simulink model "AXI_QPSK_Rx"  (R2017b)
settings: Solver=VariableStepAuto  StartTime=0.0  StopTime=2500/Rb  RelTol=1e-3
PreLoadFcn:
  | design_filters_rx;      % run script to generate filter designs.
  | 
  | Rb = 1000;   % 1kbit / s
  | 
  | Rsym = Rb/2;   % 2 bits per symbol
  | 
  | Rsymbol = Rb/2;
  | 
  | OSR = 32;
  | 
  | f_error = 120;
  | 
  | fc = 100e3;
values from neighbouring files (symbols this model uses):
  CIC_fine_Rx = 2^(-(CIC_right_shift_i-CIC_shift_Rx))    [design_filters_rx.m]
  fCIC = fCICcomp * R_CIC    (= 25600000)    [design_filters_rx.m]
  R_CIC = 3200    [design_filters_rx.m]
  R_CICcomp = 2    [design_filters_rx.m]
  R_HB = 2    [design_filters_rx.m]
  R_RRC = 4    [design_filters_rx.m]
undefined symbols (not defined in the file or in its folder): AXI4, designMultirateFIR, Lite
libraries: xbsIndex_r4 x539, dspmlti4 x12, dsparch4 x2, dspsrcs4 x2, commrandsrc2 x1, commdigbbndpm3 x1
(part 2 of 5)

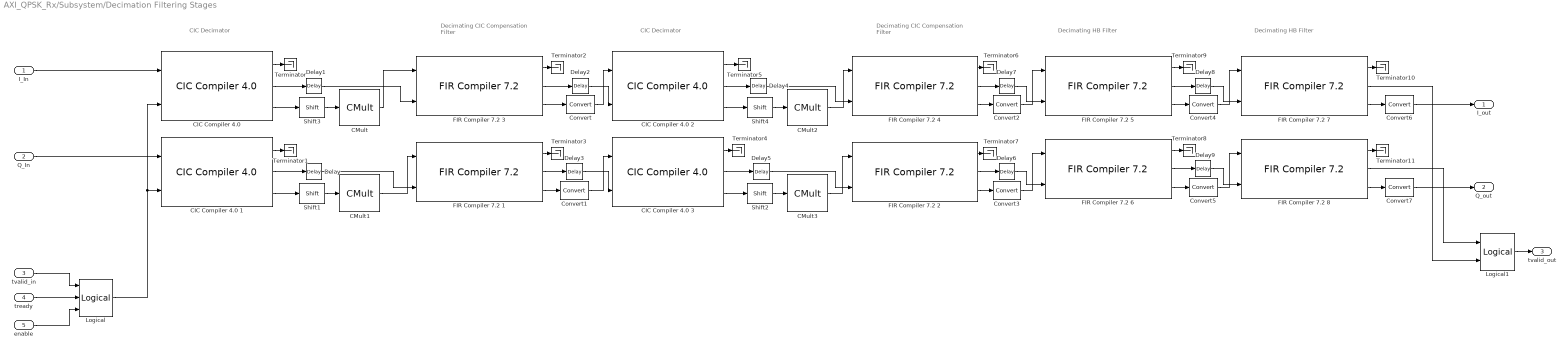
== system AXI_QPSK_Rx/Subsystem/Decimation Filtering Stages ==
  note: CIC Decimator
  note: Decimating CIC
      | Compensation Filter
  note: CIC Decimator
  note: Decimating CIC
      | Compensation Filter
  note: Decimating HB Filter
  note: Decimating HB Filter
  I_In : Inport
  Q_In : Inport  Port=2
  tvalid_in : Inport  Port=3
  tready : Inport  Port=4
  enable : Inport  Port=5
  CIC Compiler 4.0 {,1..3} (4 alike) : xbsIndex_r4/CIC Compiler 4.0   filter_type=Decimation  number_of_stages=3  differential_delay=1  number_of_channels=1  sample_rate_changes=Fixed  fixed_or_initial_rate=R_CIC_i  minimum_rate=20  maximum_rate=20  ratespecification=Maximum_Possible  sampleperiod=1  hardwareoversamplingrate=1  quantization=Full_Precision  output_data_width=31  use_xtreme_dsp_slice=on  use_streaming_interface=on  has_aclken=on  has_aresetn=off  has_dout_tready=off  trim_axipin_name=on  gui_behaviour=Sysgen_GUI  input_data_width=18  ip_name=CIC Compiler  ip_version=4.0  dsptool_ready=true  wrapper_available=true  port_translation_map={ 'aclken' => 'en', 'aresetn' => 'rst' }  ipcore_xco_need_fpga_part=true  ipcore_verbose=false  block_type=cic_compiler_v4_0
  CMult{,1..3} (4 alike) : xbsIndex_r4/CMult  const=CIC_fine_Rx  gui_display_data_type=Fixed-point  const_n_bits=16  const_bin_pt=14  float_type=Single  exp_bits=8  fraction_bits=24  en=off  latency=1  precision=User Defined  arith_type="Signed  (2's comp)"  n_bits=16  bin_pt=14  quantization=Truncate  overflow=Wrap  use_behavioral_HDL=off  mem_type=Distributed RAM  pipeline=off  dbl_ovrd=off  block_type=cmult
  Convert{,1..7} (8 alike) : xbsIndex_r4/Convert  gui_display_data_type=Fixed-point  arith_type="Signed  (2's comp)"  n_bits=16  bin_pt=14  float_type=Single  exp_bits=8  fraction_bits=24  quantization=Truncate  overflow=Wrap  en=off  latency=1  pipeline=off  dbl_ovrd=off  block_type=convert
  Delay{,1..9} (10 alike) : xbsIndex_r4/Delay  rst=off  infoeditControl=Selection of Reset will increase slice count due to use of real FFs and instead of SRLs  en=off  latency=1  reg_retiming=off  dbl_ovrd=off  block_type=delay
  FIR Compiler 7.2 {1..4} (4 alike) : xbsIndex_r4/FIR Compiler 7.2   coefficientvector=WComp_i.Numerator  coefficient_sets=1  coefficient_reload=off  filter_type=Decimation  rate_change_type=Integer  interpolation_rate=1  decimation_rate=2  zero_pack_factor=1  channel_sequence=Basic  number_channels=1  pattern_list='P4-0,P4-1,P4-2,P4-3,P4-4'  number_paths=1  ratespecification=Maximum_Possible  sampleperiod=3200  hardwareoversamplingrate=1  coefficient_sign=Signed  quantization=Quantize_Only  coefficient_width=16  bestprecision=on  coefficient_fractional_bits=15  coefficient_structure=Inferred  output_rounding_mode=Full_Precision  output_width=33  filter_architecture=Systolic_Multiply_Accumulate  optimization_goal=Area  optimization_list='None'  data_buffer_type=Automatic  coefficient_buffer_type=Automatic  input_buffer_type=Automatic  output_buffer_type=Automatic  preference_for_other_storage=Automatic  multi_column_support=Automatic  columnconfig='10'  inter_column_pipe_length=4  data_has_tlast=Not_Required  m_data_has_tready=off  s_data_has_fifo=off  s_data_has_tuser=Not_Required  m_data_has_tuser=Not_Required  s_config_sync_mode=On_Vector  s_config_method=Single  num_reload_slots=1  has_aclken=on  has_aresetn=off  infoeditControl=ARESETn must be asserted for a minimum of 2 cycles  reset_data_vector=on  trim_axipin_name=on  simulation_type=hybrid_sim  simulation_model=sysgen:xfirv7_2_cmodel  data_path_portlist={ 's_axis_data_tdata', 'm_axis_data_tdata' }  passband_min=0.0  passband_max=0.5  stopband_min=0.5  stopband_max=1.0  filter_selection=1  gui_behaviour='Sysgen_GUI'  data_sign=Signed  data_width=16  data_fractional_bits=0  data_tuser_width=1  wrapper_available=true  ip_wrap_arbitrary_binary_point=true  ip_name=FIR Compiler  ip_version=7.2  dsptool_ready=true  ipcore_usecache=true  ipcore_useipmodelcache=true  port_translation_map={ 'aclken' => 'en', 'aresetn' => 'rst' }  run_core_at_system_period=true  ipcore_xco_need_fpga_part=true  block_type=fir_compiler_v7_2
      settings: infoedit=Maximum Possible : Maximizes oversampling rate. Abstracted input handshake (no s_data_tvalid) and automatic rate propagation.<br>Hardware Oversampling Rate : Specifies oversampling rate relative to the input sample period. Abstracted input handshake (no s_data_tvalid) and automatic rate propagation.<br>Input/Output Sample Period : Specifies absolute oversampling rate. No input handshake abstraction (exposes s_data_tvalid) and no rate propagation.
  FIR Compiler 7.2 {5..8} (4 alike) : xbsIndex_r4/FIR Compiler 7.2   coefficientvector=HB.Numerator  coefficient_sets=1  coefficient_reload=off  filter_type=Decimation  rate_change_type=Integer  interpolation_rate=1  decimation_rate=2  zero_pack_factor=1  channel_sequence=Basic  number_channels=1  pattern_list='P4-0,P4-1,P4-2,P4-3,P4-4'  number_paths=1  ratespecification=Maximum_Possible  sampleperiod=3200  hardwareoversamplingrate=1  coefficient_sign=Signed  quantization=Quantize_Only  coefficient_width=16  bestprecision=on  coefficient_fractional_bits=15  coefficient_structure=Inferred  output_rounding_mode=Full_Precision  output_width=32  filter_architecture=Systolic_Multiply_Accumulate  optimization_goal=Area  optimization_list='None'  data_buffer_type=Automatic  coefficient_buffer_type=Automatic  input_buffer_type=Automatic  output_buffer_type=Automatic  preference_for_other_storage=Automatic  multi_column_support=Automatic  columnconfig='6'  inter_column_pipe_length=4  data_has_tlast=Not_Required  m_data_has_tready=off  s_data_has_fifo=off  s_data_has_tuser=Not_Required  m_data_has_tuser=Not_Required  s_config_sync_mode=On_Vector  s_config_method=Single  num_reload_slots=1  has_aclken=on  has_aresetn=off  infoeditControl=ARESETn must be asserted for a minimum of 2 cycles  reset_data_vector=on  trim_axipin_name=on  simulation_type=hybrid_sim  simulation_model=sysgen:xfirv7_2_cmodel  data_path_portlist={ 's_axis_data_tdata', 'm_axis_data_tdata' }  passband_min=0.0  passband_max=0.5  stopband_min=0.5  stopband_max=1.0  filter_selection=1  gui_behaviour='Sysgen_GUI'  data_sign=Signed  data_width=16  data_fractional_bits=0  data_tuser_width=1  wrapper_available=true  ip_wrap_arbitrary_binary_point=true  ip_name=FIR Compiler  ip_version=7.2  dsptool_ready=true  ipcore_usecache=true  ipcore_useipmodelcache=true  port_translation_map={ 'aclken' => 'en', 'aresetn' => 'rst' }  run_core_at_system_period=true  ipcore_xco_need_fpga_part=true  block_type=fir_compiler_v7_2
      settings: infoedit=Maximum Possible : Maximizes oversampling rate. Abstracted input handshake (no s_data_tvalid) and automatic rate propagation.<br>Hardware Oversampling Rate : Specifies oversampling rate relative to the input sample period. Abstracted input handshake (no s_data_tvalid) and automatic rate propagation.<br>Input/Output Sample Period : Specifies absolute oversampling rate. No input handshake abstraction (exposes s_data_tvalid) and no rate propagation.
  Logical : xbsIndex_r4/Logical  logical_function=AND  inputs=3  en=off  latency=0  precision=Full  arith_type=Unsigned  n_bits=16  bin_pt=0  align_bp=on  dbl_ovrd=off  block_type=logical
  Logical1 : xbsIndex_r4/Logical  logical_function=AND  inputs=2  en=off  latency=1  precision=Full  arith_type=Unsigned  n_bits=16  bin_pt=0  align_bp=on  dbl_ovrd=off  block_type=logical
  Shift{1..4} (4 alike) : xbsIndex_r4/Shift  shift_dir=Right  shift_bits=CIC_shift_Rx  en=off  latency=0  precision=User Defined  arith_type="Signed  (2's comp)"  n_bits=17  bin_pt=14  quantization=Truncate  overflow=Wrap  dbl_ovrd=off  block_type=shift
  Terminator{,1..11} (12 alike) : Terminator
  I_out : Outport
  Q_out : Outport  Port=2
  tvalid_out : Outport  Port=3
  wires:
  FIR Compiler 7.2 1/3 -> Convert1/1
  Shift1/1 -> CMult1/1
  CIC Compiler 4.0 1/3 -> Shift1/1
  "CIC Compiler 4.0 "/3 -> Shift3/1
  Shift3/1 -> CMult/1
  FIR Compiler 7.2 3/3 -> Convert/1
  CMult/1 -> FIR Compiler 7.2 3/1
  CMult1/1 -> FIR Compiler 7.2 1/1
  CMult3/1 -> FIR Compiler 7.2 2/1
  CMult2/1 -> FIR Compiler 7.2 4/1
  FIR Compiler 7.2 4/3 -> Convert2/1
  Shift4/1 -> CMult2/1
  CIC Compiler 4.0 2/3 -> Shift4/1
  CIC Compiler 4.0 3/3 -> Shift2/1
  Shift2/1 -> CMult3/1
  FIR Compiler 7.2 2/3 -> Convert3/1
  Convert/1 -> CIC Compiler 4.0 2/1
  Convert1/1 -> CIC Compiler 4.0 3/1
  Convert2/1 -> FIR Compiler 7.2 5/1
  Convert3/1 -> FIR Compiler 7.2 6/1
  FIR Compiler 7.2 6/3 -> Convert5/1
  FIR Compiler 7.2 5/3 -> Convert4/1
  Convert4/1 -> FIR Compiler 7.2 7/1
  Convert5/1 -> FIR Compiler 7.2 8/1
  FIR Compiler 7.2 7/3 -> Convert6/1
  FIR Compiler 7.2 8/3 -> Convert7/1
  Convert6/1 -> I_out/1
  Convert7/1 -> Q_out/1
  tready/1 -> Logical/2
  tvalid_in/1 -> Logical/1
  enable/1 -> Logical/3
  Logical/1 -> CIC Compiler 4.0 1/2, "CIC Compiler 4.0 "/2
  CIC Compiler 4.0 1/2 -> Delay/1
  Delay/1 -> FIR Compiler 7.2 1/2
  "CIC Compiler 4.0 "/2 -> Delay1/1
  Delay1/1 -> FIR Compiler 7.2 3/2
  FIR Compiler 7.2 3/2 -> Delay2/1
  Delay2/1 -> CIC Compiler 4.0 2/2
  FIR Compiler 7.2 1/2 -> Delay3/1
  Delay3/1 -> CIC Compiler 4.0 3/2
  CIC Compiler 4.0 2/2 -> Delay4/1
  Delay4/1 -> FIR Compiler 7.2 4/2
  CIC Compiler 4.0 3/2 -> Delay5/1
  Delay5/1 -> FIR Compiler 7.2 2/2
  FIR Compiler 7.2 2/2 -> Delay6/1
  Delay6/1 -> FIR Compiler 7.2 6/2
  FIR Compiler 7.2 4/2 -> Delay7/1
  Delay7/1 -> FIR Compiler 7.2 5/2
  FIR Compiler 7.2 5/2 -> Delay8/1
  Delay8/1 -> FIR Compiler 7.2 7/2
  FIR Compiler 7.2 6/2 -> Delay9/1
  Delay9/1 -> FIR Compiler 7.2 8/2
  Logical1/1 -> tvalid_out/1
  "CIC Compiler 4.0 "/1 -> Terminator/1
  CIC Compiler 4.0 1/1 -> Terminator1/1
  FIR Compiler 7.2 3/1 -> Terminator2/1
  FIR Compiler 7.2 1/1 -> Terminator3/1
  CIC Compiler 4.0 3/1 -> Terminator4/1
  CIC Compiler 4.0 2/1 -> Terminator5/1
  FIR Compiler 7.2 4/1 -> Terminator6/1
  FIR Compiler 7.2 2/1 -> Terminator7/1
  FIR Compiler 7.2 6/1 -> Terminator8/1
  FIR Compiler 7.2 5/1 -> Terminator9/1
  FIR Compiler 7.2 7/1 -> Terminator10/1
  FIR Compiler 7.2 8/2 -> Logical1/1
  FIR Compiler 7.2 7/2 -> Logical1/2
  FIR Compiler 7.2 8/1 -> Terminator11/1
  I_In/1 -> "CIC Compiler 4.0 "/1
  Q_In/1 -> CIC Compiler 4.0 1/1

== system AXI_QPSK_Rx/Subsystem/M_AXIS ==
  tData_in : Inport
  tValid_in : Inport  Port=2
  tLast_in : Inport  Port=3
  tReady_in : Inport  Port=4
  m_rf_axis_tdata : xbsIndex_r4/Gateway Out  inherit_from_input=off  hdl_port=on  rows=1  columns=1  UseAsDAC=off  DACChannel='1'  interface=None  automatic_assignment=on  address_offset=hex2dec('00')  intf_name=''  intf_description=''  timing_constraint=None  locs_specified=off  LOCs={}  io_standard={}  block_type=gatewayout
  m_rf_axis_tlast : xbsIndex_r4/Gateway Out  inherit_from_input=off  hdl_port=on  rows=1  columns=1  UseAsDAC=off  DACChannel='1'  interface=None  automatic_assignment=on  address_offset=hex2dec('00')  intf_name=''  intf_description=''  timing_constraint=None  locs_specified=off  LOCs={}  io_standard={}  block_type=gatewayout
  m_rf_axis_tready : xbsIndex_r4/Gateway In  gui_display_data_type=Boolean  arith_type=Boolean  n_bits=16  bin_pt=14  preci_type=Single  exp_width=8  frac_width=24  rows=1  columns=1  quantization="Round  (unbiased: +/- Inf)"  overflow=Saturate  period=1/(0.5*R_RRC*R_HB*R_CICcomp*R_CIC*Rb)  UseAsADC=off  ADCChannel='1'  interface=None  automatic_assignment=on  address_offset=hex2dec('00')  intf_name=''  intf_description=''  default_value=0  timing_constraint=None  locs_specified=off  LOCs={}  io_standard={}  inherit_from_input=off  hdl_port=on  dbl_ovrd=off  block_type=gatewayin
  m_rf_axis_tvalid : xbsIndex_r4/Gateway Out  inherit_from_input=off  hdl_port=on  rows=1  columns=1  UseAsDAC=off  DACChannel='1'  interface=None  automatic_assignment=on  address_offset=hex2dec('00')  intf_name=''  intf_description=''  timing_constraint=None  locs_specified=off  LOCs={}  io_standard={}  block_type=gatewayout
  tData_out : Outport
  tLast_out : Outport  Port=2
  tValid_out : Outport  Port=3
  tReady_out : Outport  Port=4
  wires:
  tReady_in/1 -> m_rf_axis_tready/1
  m_rf_axis_tlast/1 -> tLast_out/1
  m_rf_axis_tvalid/1 -> tValid_out/1
  m_rf_axis_tdata/1 -> tData_out/1
  tData_in/1 -> m_rf_axis_tdata/1
  tLast_in/1 -> m_rf_axis_tlast/1
  tValid_in/1 -> m_rf_axis_tvalid/1
  m_rf_axis_tready/1 -> tReady_out/1

== system AXI_QPSK_Rx/Subsystem/M_AXIS_DECIMATION ==
  tData_in : Inport
  tValid_in : Inport  Port=2
  tLast_in : Inport  Port=3
  tReady_in : Inport  Port=4
  m_dec_axis_tdata : xbsIndex_r4/Gateway Out  inherit_from_input=off  hdl_port=on  rows=1  columns=1  UseAsDAC=off  DACChannel='1'  interface=None  automatic_assignment=on  address_offset=hex2dec('00')  intf_name=''  intf_description=''  timing_constraint=None  locs_specified=off  LOCs={}  io_standard={}  block_type=gatewayout
  m_dec_axis_tlast : xbsIndex_r4/Gateway Out  inherit_from_input=off  hdl_port=on  rows=1  columns=1  UseAsDAC=off  DACChannel='1'  interface=None  automatic_assignment=on  address_offset=hex2dec('00')  intf_name=''  intf_description=''  timing_constraint=None  locs_specified=off  LOCs={}  io_standard={}  block_type=gatewayout
  m_dec_axis_tready : xbsIndex_r4/Gateway In  gui_display_data_type=Boolean  arith_type=Boolean  n_bits=16  bin_pt=14  preci_type=Single  exp_width=8  frac_width=24  rows=1  columns=1  quantization="Round  (unbiased: +/- Inf)"  overflow=Saturate  period=1/(0.5*R_RRC*R_HB*R_CICcomp*R_CIC*Rb)  UseAsADC=off  ADCChannel='1'  interface=None  automatic_assignment=on  address_offset=hex2dec('00')  intf_name=''  intf_description=''  default_value=0  timing_constraint=None  locs_specified=off  LOCs={}  io_standard={}  inherit_from_input=off  hdl_port=on  dbl_ovrd=off  block_type=gatewayin
  m_dec_axis_tvalid : xbsIndex_r4/Gateway Out  inherit_from_input=off  hdl_port=on  rows=1  columns=1  UseAsDAC=off  DACChannel='1'  interface=None  automatic_assignment=on  address_offset=hex2dec('00')  intf_name=''  intf_description=''  timing_constraint=None  locs_specified=off  LOCs={}  io_standard={}  block_type=gatewayout
  tData_out : Outport
  tLast_out : Outport  Port=2
  tValid_out : Outport  Port=3
  tReady_out : Outport  Port=4
  wires:
  m_dec_axis_tready/1 -> tReady_out/1
  tValid_in/1 -> m_dec_axis_tvalid/1
  tLast_in/1 -> m_dec_axis_tlast/1
  tData_in/1 -> m_dec_axis_tdata/1
  m_dec_axis_tdata/1 -> tData_out/1
  m_dec_axis_tvalid/1 -> tValid_out/1
  m_dec_axis_tlast/1 -> tLast_out/1
  tReady_in/1 -> m_dec_axis_tready/1

== system AXI_QPSK_Rx/Subsystem/M_AXIS_FREQ_SYNC ==
  tData_in : Inport
  tValid_in : Inport  Port=2
  tLast_in : Inport  Port=3
  tReady_in : Inport  Port=4
  m_sync_axis_tdata : xbsIndex_r4/Gateway Out  inherit_from_input=off  hdl_port=on  rows=1  columns=1  UseAsDAC=off  DACChannel='1'  interface=None  automatic_assignment=on  address_offset=hex2dec('00')  intf_name=''  intf_description=''  timing_constraint=None  locs_specified=off  LOCs={}  io_standard={}  block_type=gatewayout
  m_sync_axis_tlast : xbsIndex_r4/Gateway Out  inherit_from_input=off  hdl_port=on  rows=1  columns=1  UseAsDAC=off  DACChannel='1'  interface=None  automatic_assignment=on  address_offset=hex2dec('00')  intf_name=''  intf_description=''  timing_constraint=None  locs_specified=off  LOCs={}  io_standard={}  block_type=gatewayout
  m_sync_axis_tready : xbsIndex_r4/Gateway In  gui_display_data_type=Boolean  arith_type=Boolean  n_bits=16  bin_pt=14  preci_type=Single  exp_width=8  frac_width=24  rows=1  columns=1  quantization="Round  (unbiased: +/- Inf)"  overflow=Saturate  period=1/(0.5*R_RRC*R_HB*R_CICcomp*R_CIC*Rb)  UseAsADC=off  ADCChannel='1'  interface=None  automatic_assignment=on  address_offset=hex2dec('00')  intf_name=''  intf_description=''  default_value=0  timing_constraint=None  locs_specified=off  LOCs={}  io_standard={}  inherit_from_input=off  hdl_port=on  dbl_ovrd=off  block_type=gatewayin
  m_sync_axis_tvalid : xbsIndex_r4/Gateway Out  inherit_from_input=off  hdl_port=on  rows=1  columns=1  UseAsDAC=off  DACChannel='1'  interface=None  automatic_assignment=on  address_offset=hex2dec('00')  intf_name=''  intf_description=''  timing_constraint=None  locs_specified=off  LOCs={}  io_standard={}  block_type=gatewayout
  tData_out : Outport
  tLast_out : Outport  Port=2
  tValid_out : Outport  Port=3
  tReady_out : Outport  Port=4
  wires:
  tReady_in/1 -> m_sync_axis_tready/1
  m_sync_axis_tlast/1 -> tLast_out/1
  m_sync_axis_tvalid/1 -> tValid_out/1
  m_sync_axis_tdata/1 -> tData_out/1
  tData_in/1 -> m_sync_axis_tdata/1
  tLast_in/1 -> m_sync_axis_tlast/1
  tValid_in/1 -> m_sync_axis_tvalid/1
  m_sync_axis_tready/1 -> tReady_out/1

== system AXI_QPSK_Rx/Subsystem/M_AXIS_RRC ==
  tData_in : Inport
  tValid_in : Inport  Port=2
  tLast_in : Inport  Port=3
  tReady_in : Inport  Port=4
  m_rrc_axis_tdata : xbsIndex_r4/Gateway Out  inherit_from_input=off  hdl_port=on  rows=1  columns=1  UseAsDAC=off  DACChannel='1'  interface=None  automatic_assignment=on  address_offset=hex2dec('00')  intf_name=''  intf_description=''  timing_constraint=None  locs_specified=off  LOCs={}  io_standard={}  block_type=gatewayout
  m_rrc_axis_tlast : xbsIndex_r4/Gateway Out  inherit_from_input=off  hdl_port=on  rows=1  columns=1  UseAsDAC=off  DACChannel='1'  interface=None  automatic_assignment=on  address_offset=hex2dec('00')  intf_name=''  intf_description=''  timing_constraint=None  locs_specified=off  LOCs={}  io_standard={}  block_type=gatewayout
  m_rrc_axis_tready : xbsIndex_r4/Gateway In  gui_display_data_type=Boolean  arith_type=Boolean  n_bits=16  bin_pt=14  preci_type=Single  exp_width=8  frac_width=24  rows=1  columns=1  quantization="Round  (unbiased: +/- Inf)"  overflow=Saturate  period=1/(0.5*R_RRC*R_HB*R_CICcomp*R_CIC*Rb)  UseAsADC=off  ADCChannel='1'  interface=None  automatic_assignment=on  address_offset=hex2dec('00')  intf_name=''  intf_description=''  default_value=0  timing_constraint=None  locs_specified=off  LOCs={}  io_standard={}  inherit_from_input=off  hdl_port=on  dbl_ovrd=off  block_type=gatewayin
  m_rrc_axis_tvalid : xbsIndex_r4/Gateway Out  inherit_from_input=off  hdl_port=on  rows=1  columns=1  UseAsDAC=off  DACChannel='1'  interface=None  automatic_assignment=on  address_offset=hex2dec('00')  intf_name=''  intf_description=''  timing_constraint=None  locs_specified=off  LOCs={}  io_standard={}  block_type=gatewayout
  tData_out : Outport
  tLast_out : Outport  Port=2
  tValid_out : Outport  Port=3
  tReady_out : Outport  Port=4
  wires:
  tReady_in/1 -> m_rrc_axis_tready/1
  m_rrc_axis_tlast/1 -> tLast_out/1
  m_rrc_axis_tvalid/1 -> tValid_out/1
  m_rrc_axis_tdata/1 -> tData_out/1
  tData_in/1 -> m_rrc_axis_tdata/1
  tLast_in/1 -> m_rrc_axis_tlast/1
  tValid_in/1 -> m_rrc_axis_tvalid/1
  m_rrc_axis_tready/1 -> tReady_out/1

== system AXI_QPSK_Rx/Subsystem/RRC Filtering and Pre-Synch Interpolation  ==
  note: Root Raised Cosine Receive Filter
      | (single rate)
  note: Interpolating (x2) Halfband Filter
  note: Interpolating (x2) Halfband Filter
  I_in : Inport
  Q_in : Inport  Port=2
  tvalid_in : Inport  Port=3
  Delay{1..4} (4 alike) : xbsIndex_r4/Delay  rst=off  infoeditControl=Selection of Reset will increase slice count due to use of real FFs and instead of SRLs  en=off  latency=1  reg_retiming=off  dbl_ovrd=off  block_type=delay
  FIR Compiler 7.2 2 : xbsIndex_r4/FIR Compiler 7.2   coefficientvector=WRRC2.Numerator  coefficient_sets=1  coefficient_reload=off  filter_type=Single_Rate  rate_change_type=Integer  interpolation_rate=1  decimation_rate=1  zero_pack_factor=1  channel_sequence=Basic  number_channels=1  pattern_list='P4-0,P4-1,P4-2,P4-3,P4-4'  number_paths=1  ratespecification=Maximum_Possible  sampleperiod=1  hardwareoversamplingrate=1  coefficient_sign=Signed  quantization=Quantize_Only  coefficient_width=16  bestprecision=on  coefficient_fractional_bits=16  coefficient_structure=Inferred  output_rounding_mode=Full_Precision  output_width=35  filter_architecture=Systolic_Multiply_Accumulate  optimization_goal=Area  optimization_list='None'  data_buffer_type=Automatic  coefficient_buffer_type=Automatic  input_buffer_type=Automatic  output_buffer_type=Automatic  preference_for_other_storage=Automatic  multi_column_support=Automatic  columnconfig='49'  inter_column_pipe_length=4  data_has_tlast=Not_Required  m_data_has_tready=off  s_data_has_fifo=off  s_data_has_tuser=Not_Required  m_data_has_tuser=Not_Required  s_config_sync_mode=On_Vector  s_config_method=Single  num_reload_slots=1  has_aclken=on  has_aresetn=off  infoeditControl=ARESETn must be asserted for a minimum of 2 cycles  reset_data_vector=on  trim_axipin_name=on  simulation_type=hybrid_sim  simulation_model=sysgen:xfirv7_2_cmodel  data_path_portlist={ 's_axis_data_tdata', 'm_axis_data_tdata' }  passband_min=0.0  passband_max=0.5  stopband_min=0.5  stopband_max=1.0  filter_selection=1  gui_behaviour='Sysgen_GUI'  data_sign=Signed  data_width=16  data_fractional_bits=0  data_tuser_width=1  wrapper_available=true  ip_wrap_arbitrary_binary_point=true  ip_name=FIR Compiler  ip_version=7.2  dsptool_ready=true  ipcore_usecache=true  ipcore_useipmodelcache=true  port_translation_map={ 'aclken' => 'en', 'aresetn' => 'rst' }  run_core_at_system_period=true  ipcore_xco_need_fpga_part=true  block_type=fir_compiler_v7_2
      settings: infoedit=Maximum Possible : Maximizes oversampling rate. Abstracted input handshake (no s_data_tvalid) and automatic rate propagation.<br>Hardware Oversampling Rate : Specifies oversampling rate relative to the input sample period. Abstracted input handshake (no s_data_tvalid) and automatic rate propagation.<br>Input/Output Sample Period : Specifies absolute oversampling rate. No input handshake abstraction (exposes s_data_tvalid) and no rate propagation.
  FIR Compiler 7.2 4 : xbsIndex_r4/FIR Compiler 7.2   coefficientvector=WRRC2.Numerator  coefficient_sets=1  coefficient_reload=off  filter_type=Single_Rate  rate_change_type=Integer  interpolation_rate=1  decimation_rate=1  zero_pack_factor=1  channel_sequence=Basic  number_channels=1  pattern_list='P4-0,P4-1,P4-2,P4-3,P4-4'  number_paths=1  ratespecification=Maximum_Possible  sampleperiod=1  hardwareoversamplingrate=1  coefficient_sign=Signed  quantization=Quantize_Only  coefficient_width=16  bestprecision=on  coefficient_fractional_bits=16  coefficient_structure=Inferred  output_rounding_mode=Full_Precision  output_width=35  filter_architecture=Systolic_Multiply_Accumulate  optimization_goal=Area  optimization_list='None'  data_buffer_type=Automatic  coefficient_buffer_type=Automatic  input_buffer_type=Automatic  output_buffer_type=Automatic  preference_for_other_storage=Automatic  multi_column_support=Automatic  columnconfig='49'  inter_column_pipe_length=4  data_has_tlast=Not_Required  m_data_has_tready=off  s_data_has_fifo=off  s_data_has_tuser=Not_Required  m_data_has_tuser=Not_Required  s_config_sync_mode=On_Vector  s_config_method=Single  num_reload_slots=1  has_aclken=on  has_aresetn=off  infoeditControl=ARESETn must be asserted for a minimum of 2 cycles  reset_data_vector=on  trim_axipin_name=on  simulation_type=hybrid_sim  simulation_model=sysgen:xfirv7_2_cmodel  data_path_portlist={ 's_axis_data_tdata', 'm_axis_data_tdata' }  passband_min=0.0  passband_max=0.5  stopband_min=0.5  stopband_max=1.0  filter_selection=1  gui_behaviour='Sysgen_GUI'  data_sign=Signed  data_width=16  data_fractional_bits=0  data_tuser_width=1  wrapper_available=true  ip_wrap_arbitrary_binary_point=true  ip_name=FIR Compiler  ip_version=7.2  dsptool_ready=true  ipcore_usecache=true  ipcore_useipmodelcache=true  port_translation_map={ 'aclken' => 'en', 'aresetn' => 'rst' }  run_core_at_system_period=true  ipcore_xco_need_fpga_part=true  block_type=fir_compiler_v7_2
      settings: infoedit=Maximum Possible : Maximizes oversampling rate. Abstracted input handshake (no s_data_tvalid) and automatic rate propagation.<br>Hardware Oversampling Rate : Specifies oversampling rate relative to the input sample period. Abstracted input handshake (no s_data_tvalid) and automatic rate propagation.<br>Input/Output Sample Period : Specifies absolute oversampling rate. No input handshake abstraction (exposes s_data_tvalid) and no rate propagation.
  FIR Compiler 7.2 {5..8} (4 alike) : xbsIndex_r4/FIR Compiler 7.2   coefficientvector=HB.Numerator  coefficient_sets=1  coefficient_reload=off  filter_type=Interpolation  rate_change_type=Integer  interpolation_rate=2  decimation_rate=1  zero_pack_factor=1  channel_sequence=Basic  number_channels=1  pattern_list='P4-0,P4-1,P4-2,P4-3,P4-4'  number_paths=1  ratespecification=Maximum_Possible  sampleperiod=1  hardwareoversamplingrate=1  coefficient_sign=Signed  quantization=Quantize_Only  coefficient_width=16  bestprecision=on  coefficient_fractional_bits=15  coefficient_structure=Inferred  output_rounding_mode=Full_Precision  output_width=32  filter_architecture=Systolic_Multiply_Accumulate  optimization_goal=Area  optimization_list='None'  data_buffer_type=Automatic  coefficient_buffer_type=Automatic  input_buffer_type=Automatic  output_buffer_type=Automatic  preference_for_other_storage=Automatic  multi_column_support=Automatic  columnconfig='24'  inter_column_pipe_length=4  data_has_tlast=Not_Required  m_data_has_tready=off  s_data_has_fifo=off  s_data_has_tuser=Not_Required  m_data_has_tuser=Not_Required  s_config_sync_mode=On_Vector  s_config_method=Single  num_reload_slots=1  has_aclken=on  has_aresetn=off  infoeditControl=ARESETn must be asserted for a minimum of 2 cycles  reset_data_vector=on  trim_axipin_name=on  simulation_type=hybrid_sim  simulation_model=sysgen:xfirv7_2_cmodel  data_path_portlist={ 's_axis_data_tdata', 'm_axis_data_tdata' }  passband_min=0.0  passband_max=0.5  stopband_min=0.5  stopband_max=1.0  filter_selection=1  gui_behaviour='Sysgen_GUI'  data_sign=Signed  data_width=16  data_fractional_bits=0  data_tuser_width=1  wrapper_available=true  ip_wrap_arbitrary_binary_point=true  ip_name=FIR Compiler  ip_version=7.2  dsptool_ready=true  ipcore_usecache=true  ipcore_useipmodelcache=true  port_translation_map={ 'aclken' => 'en', 'aresetn' => 'rst' }  run_core_at_system_period=true  ipcore_xco_need_fpga_part=true  block_type=fir_compiler_v7_2
      settings: infoedit=Maximum Possible : Maximizes oversampling rate. Abstracted input handshake (no s_data_tvalid) and automatic rate propagation.<br>Hardware Oversampling Rate : Specifies oversampling rate relative to the input sample period. Abstracted input handshake (no s_data_tvalid) and automatic rate propagation.<br>Input/Output Sample Period : Specifies absolute oversampling rate. No input handshake abstraction (exposes s_data_tvalid) and no rate propagation.
  Logical : xbsIndex_r4/Logical  logical_function=AND  inputs=2  en=off  latency=1  precision=Full  arith_type=Unsigned  n_bits=16  bin_pt=0  align_bp=on  dbl_ovrd=off  block_type=logical
  Shift : xbsIndex_r4/Shift  shift_dir=Right  shift_bits=1  en=off  latency=1  precision=User Defined  arith_type="Signed  (2's comp)"  n_bits=16  bin_pt=14  quantization=Truncate  overflow=Wrap  dbl_ovrd=off  block_type=shift
  Shift2 : xbsIndex_r4/Shift  shift_dir=Right  shift_bits=1  en=off  latency=1  precision=User Defined  arith_type="Signed  (2's comp)"  n_bits=16  bin_pt=14  quantization=Truncate  overflow=Wrap  dbl_ovrd=off  block_type=shift
  Shift{4..7} (4 alike) : xbsIndex_r4/Shift  shift_dir=Left  shift_bits=1  en=off  latency=1  precision=User Defined  arith_type="Signed  (2's comp)"  n_bits=16  bin_pt=14  quantization=Truncate  overflow=Wrap  dbl_ovrd=off  block_type=shift
  I_out : Outport
  Q_out : Outport  Port=2
  tvalid_out : Outport  Port=3
  wires:
  Shift7/1 -> Q_out/1
  Shift6/1 -> I_out/1
  Shift5/1 -> FIR Compiler 7.2 8/1
  Shift4/1 -> FIR Compiler 7.2 7/1
  FIR Compiler 7.2 7/3 -> Shift6/1
  FIR Compiler 7.2 8/3 -> Shift7/1
  FIR Compiler 7.2 6/3 -> Shift5/1
  Q_in/1 -> FIR Compiler 7.2 4/1
  FIR Compiler 7.2 5/3 -> Shift4/1
  FIR Compiler 7.2 4/3 -> Shift2/1
  I_in/1 -> FIR Compiler 7.2 2/1
  FIR Compiler 7.2 2/3 -> Shift/1
  Shift2/1 -> FIR Compiler 7.2 6/1
  Shift/1 -> FIR Compiler 7.2 5/1
  tvalid_in/1 -> FIR Compiler 7.2 4/2, FIR Compiler 7.2 2/2
  FIR Compiler 7.2 4/2 -> Delay1/1
  FIR Compiler 7.2 2/2 -> Delay2/1
  Delay1/1 -> FIR Compiler 7.2 6/2
  Delay2/1 -> FIR Compiler 7.2 5/2
  FIR Compiler 7.2 6/2 -> Delay4/1
  FIR Compiler 7.2 5/2 -> Delay3/1
  Logical/1 -> tvalid_out/1
  FIR Compiler 7.2 7/2 -> Logical/1
  FIR Compiler 7.2 8/2 -> Logical/2
  Delay3/1 -> FIR Compiler 7.2 7/2
  Delay4/1 -> FIR Compiler 7.2 8/2

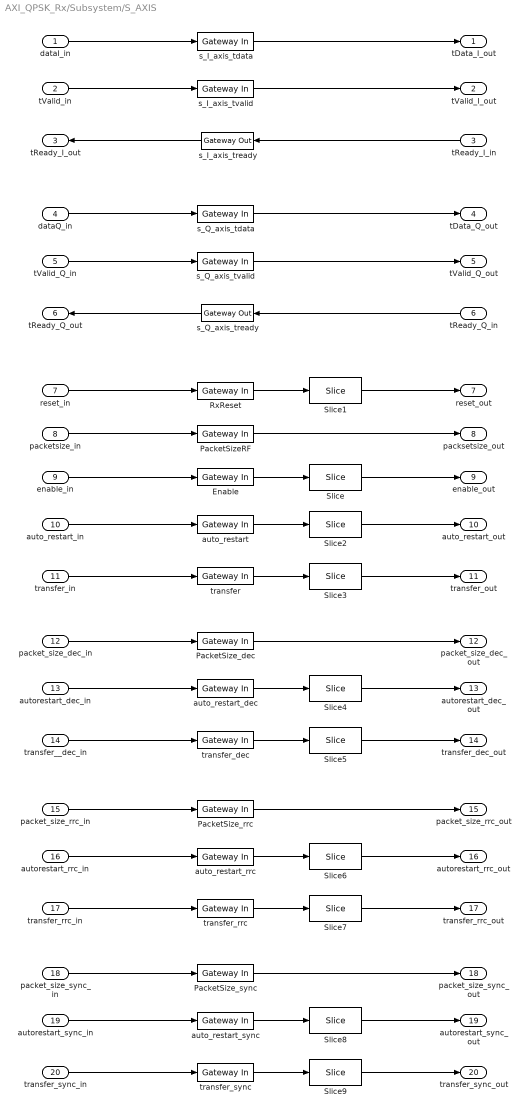
== system AXI_QPSK_Rx/Subsystem/S_AXIS ==
  dataI_in : Inport
  tValid_in : Inport  Port=2
  tReady_I_in : Inport  Port=3
  dataQ_in : Inport  Port=4
  tValid_Q_in : Inport  Port=5
  tReady_Q_in : Inport  Port=6
  reset_in : Inport  Port=7
  packetsize_in : Inport  Port=8
  enable_in : Inport  Port=9
  auto_restart_in : Inport  Port=10
  transfer_in : Inport  Port=11
  packet_size_dec_in : Inport  Port=12
  autorestart_dec_in : Inport  Port=13
  transfer__dec_in : Inport  Port=14
  packet_size_rrc_in : Inport  Port=15
  autorestart_rrc_in : Inport  Port=16
  transfer_rrc_in : Inport  Port=17
  packet_size_sync_in : Inport  Port=18
  autorestart_sync_in : Inport  Port=19
  transfer_sync_in : Inport  Port=20
  Enable : xbsIndex_r4/Gateway In  gui_display_data_type=Fixed-point  arith_type=Unsigned  n_bits=32  bin_pt=0  preci_type=Single  exp_width=8  frac_width=24  rows=1  columns=1  quantization="Round  (unbiased: +/- Inf)"  overflow=Saturate  period=1/(0.5*R_RRC*R_HB*R_CICcomp*R_CIC*Rb)  UseAsADC=off  ADCChannel='1'  interface=AXI4-Lite  automatic_assignment=off  address_offset=32  intf_name=''  intf_description=''  default_value=0  timing_constraint=None  locs_specified=off  LOCs={}  io_standard={}  inherit_from_input=off  hdl_port=on  dbl_ovrd=off  block_type=gatewayin
  PacketSizeRF : xbsIndex_r4/Gateway In  gui_display_data_type=Fixed-point  arith_type=Unsigned  n_bits=32  bin_pt=0  preci_type=Single  exp_width=8  frac_width=24  rows=1  columns=1  quantization=Truncate  overflow=Wrap  period=1/(0.5*R_RRC*R_HB*R_CICcomp*R_CIC*Rb)  UseAsADC=off  ADCChannel='1'  interface=AXI4-Lite  automatic_assignment=off  address_offset=20  intf_name=''  intf_description=''  default_value=0  timing_constraint=None  locs_specified=off  LOCs={}  io_standard={}  inherit_from_input=off  hdl_port=on  dbl_ovrd=off  block_type=gatewayin
  PacketSize_dec : xbsIndex_r4/Gateway In  gui_display_data_type=Fixed-point  arith_type=Unsigned  n_bits=32  bin_pt=0  preci_type=Single  exp_width=8  frac_width=24  rows=1  columns=1  quantization=Truncate  overflow=Wrap  period=1/(0.5*R_RRC*R_HB*R_CICcomp*R_CIC*Rb)  UseAsADC=off  ADCChannel='1'  interface=AXI4-Lite  automatic_assignment=off  address_offset=44  intf_name=''  intf_description=''  default_value=0  timing_constraint=None  locs_specified=off  LOCs={}  io_standard={}  inherit_from_input=off  hdl_port=on  dbl_ovrd=off  block_type=gatewayin
  PacketSize_rrc : xbsIndex_r4/Gateway In  gui_display_data_type=Fixed-point  arith_type=Unsigned  n_bits=32  bin_pt=0  preci_type=Single  exp_width=8  frac_width=24  rows=1  columns=1  quantization=Truncate  overflow=Wrap  period=1/(0.5*R_RRC*R_HB*R_CICcomp*R_CIC*Rb)  UseAsADC=off  ADCChannel='1'  interface=AXI4-Lite  automatic_assignment=off  address_offset=56  intf_name=''  intf_description=''  default_value=0  timing_constraint=None  locs_specified=off  LOCs={}  io_standard={}  inherit_from_input=off  hdl_port=on  dbl_ovrd=off  block_type=gatewayin
  PacketSize_sync : xbsIndex_r4/Gateway In  gui_display_data_type=Fixed-point  arith_type=Unsigned  n_bits=32  bin_pt=0  preci_type=Single  exp_width=8  frac_width=24  rows=1  columns=1  quantization=Truncate  overflow=Wrap  period=1/(0.5*R_RRC*R_HB*R_CICcomp*R_CIC*Rb)  UseAsADC=off  ADCChannel='1'  interface=AXI4-Lite  automatic_assignment=off  address_offset=68  intf_name=''  intf_description=''  default_value=0  timing_constraint=None  locs_specified=off  LOCs={}  io_standard={}  inherit_from_input=off  hdl_port=on  dbl_ovrd=off  block_type=gatewayin
  RxReset : xbsIndex_r4/Gateway In  gui_display_data_type=Fixed-point  arith_type=Unsigned  n_bits=32  bin_pt=0  preci_type=Single  exp_width=8  frac_width=24  rows=1  columns=1  quantization="Round  (unbiased: +/- Inf)"  overflow=Saturate  period=1/(0.5*R_RRC*R_HB*R_CICcomp*R_CIC*Rb)  UseAsADC=off  ADCChannel='1'  interface=AXI4-Lite  automatic_assignment=off  address_offset=28  intf_name=''  intf_description=''  default_value=0  timing_constraint=None  locs_specified=off  LOCs={}  io_standard={}  inherit_from_input=off  hdl_port=on  dbl_ovrd=off  block_type=gatewayin
  Slice{,1..9} (10 alike) : xbsIndex_r4/Slice  nbits=1  boolean_output=on  mode=Two Bit Locations  bit1=0  base1=LSB of Input  bit0=0  base0=LSB of Input  dbl_ovrd=off  block_type=slice
  auto_restart : xbsIndex_r4/Gateway In  gui_display_data_type=Fixed-point  arith_type=Unsigned  n_bits=32  bin_pt=0  preci_type=Single  exp_width=8  frac_width=24  rows=1  columns=1  quantization="Round  (unbiased: +/- Inf)"  overflow=Saturate  period=1/(0.5*R_RRC*R_HB*R_CICcomp*R_CIC*Rb)  UseAsADC=off  ADCChannel='1'  interface=AXI4-Lite  automatic_assignment=off  address_offset=36  intf_name=''  intf_description=''  default_value=0  timing_constraint=None  locs_specified=off  LOCs={}  io_standard={}  inherit_from_input=off  hdl_port=on  dbl_ovrd=off  block_type=gatewayin
  auto_restart_dec : xbsIndex_r4/Gateway In  gui_display_data_type=Fixed-point  arith_type=Unsigned  n_bits=32  bin_pt=0  preci_type=Single  exp_width=8  frac_width=24  rows=1  columns=1  quantization="Round  (unbiased: +/- Inf)"  overflow=Saturate  period=1/(0.5*R_RRC*R_HB*R_CICcomp*R_CIC*Rb)  UseAsADC=off  ADCChannel='1'  interface=AXI4-Lite  automatic_assignment=off  address_offset=48  intf_name=''  intf_description=''  default_value=0  timing_constraint=None  locs_specified=off  LOCs={}  io_standard={}  inherit_from_input=off  hdl_port=on  dbl_ovrd=off  block_type=gatewayin
  auto_restart_rrc : xbsIndex_r4/Gateway In  gui_display_data_type=Fixed-point  arith_type=Unsigned  n_bits=32  bin_pt=0  preci_type=Single  exp_width=8  frac_width=24  rows=1  columns=1  quantization="Round  (unbiased: +/- Inf)"  overflow=Saturate  period=1/(0.5*R_RRC*R_HB*R_CICcomp*R_CIC*Rb)  UseAsADC=off  ADCChannel='1'  interface=AXI4-Lite  automatic_assignment=off  address_offset=60  intf_name=''  intf_description=''  default_value=0  timing_constraint=None  locs_specified=off  LOCs={}  io_standard={}  inherit_from_input=off  hdl_port=on  dbl_ovrd=off  block_type=gatewayin
  auto_restart_sync : xbsIndex_r4/Gateway In  gui_display_data_type=Fixed-point  arith_type=Unsigned  n_bits=32  bin_pt=0  preci_type=Single  exp_width=8  frac_width=24  rows=1  columns=1  quantization="Round  (unbiased: +/- Inf)"  overflow=Saturate  period=1/(0.5*R_RRC*R_HB*R_CICcomp*R_CIC*Rb)  UseAsADC=off  ADCChannel='1'  interface=AXI4-Lite  automatic_assignment=off  address_offset=72  intf_name=''  intf_description=''  default_value=0  timing_constraint=None  locs_specified=off  LOCs={}  io_standard={}  inherit_from_input=off  hdl_port=on  dbl_ovrd=off  block_type=gatewayin
  s_I_axis_tdata : xbsIndex_r4/Gateway In  gui_display_data_type=Fixed-point  arith_type="Signed  (2's comp)"  n_bits=16  bin_pt=14  preci_type=Single  exp_width=8  frac_width=24  rows=1  columns=1  quantization="Round  (unbiased: +/- Inf)"  overflow=Saturate  period=1/(0.5*R_RRC*R_HB*R_CICcomp*R_CIC*Rb)  UseAsADC=off  ADCChannel='1'  interface=None  automatic_assignment=on  address_offset=hex2dec('00')  intf_name=''  intf_description=''  default_value=0  timing_constraint=None  locs_specified=off  LOCs={}  io_standard={}  inherit_from_input=off  hdl_port=on  dbl_ovrd=off  block_type=gatewayin
  s_I_axis_tready : xbsIndex_r4/Gateway Out  inherit_from_input=off  hdl_port=on  rows=1  columns=1  UseAsDAC=off  DACChannel='1'  interface=None  automatic_assignment=on  address_offset=hex2dec('00')  intf_name=''  intf_description=''  timing_constraint=None  locs_specified=off  LOCs={}  io_standard={}  block_type=gatewayout
  s_I_axis_tvalid : xbsIndex_r4/Gateway In  gui_display_data_type=Boolean  arith_type=Boolean  n_bits=32  bin_pt=0  preci_type=Single  exp_width=8  frac_width=24  rows=1  columns=1  quantization="Round  (unbiased: +/- Inf)"  overflow=Saturate  period=1/(0.5*R_RRC*R_HB*R_CICcomp*R_CIC*Rb)  UseAsADC=off  ADCChannel='1'  interface=None  automatic_assignment=on  address_offset=hex2dec('00')  intf_name=''  intf_description=''  default_value=0  timing_constraint=None  locs_specified=off  LOCs={}  io_standard={}  inherit_from_input=off  hdl_port=on  dbl_ovrd=off  block_type=gatewayin
  s_Q_axis_tdata : xbsIndex_r4/Gateway In  gui_display_data_type=Fixed-point  arith_type="Signed  (2's comp)"  n_bits=16  bin_pt=14  preci_type=Single  exp_width=8  frac_width=24  rows=1  columns=1  quantization="Round  (unbiased: +/- Inf)"  overflow=Saturate  period=1/(0.5*R_RRC*R_HB*R_CICcomp*R_CIC*Rb)  UseAsADC=off  ADCChannel='1'  interface=None  automatic_assignment=on  address_offset=hex2dec('00')  intf_name=''  intf_description=''  default_value=0  timing_constraint=None  locs_specified=off  LOCs={}  io_standard={}  inherit_from_input=off  hdl_port=on  dbl_ovrd=off  block_type=gatewayin
  s_Q_axis_tready : xbsIndex_r4/Gateway Out  inherit_from_input=off  hdl_port=on  rows=1  columns=1  UseAsDAC=off  DACChannel='1'  interface=None  automatic_assignment=on  address_offset=hex2dec('00')  intf_name=''  intf_description=''  timing_constraint=None  locs_specified=off  LOCs={}  io_standard={}  block_type=gatewayout
  s_Q_axis_tvalid : xbsIndex_r4/Gateway In  gui_display_data_type=Boolean  arith_type=Boolean  n_bits=32  bin_pt=0  preci_type=Single  exp_width=8  frac_width=24  rows=1  columns=1  quantization="Round  (unbiased: +/- Inf)"  overflow=Saturate  period=1/(0.5*R_RRC*R_HB*R_CICcomp*R_CIC*Rb)  UseAsADC=off  ADCChannel='1'  interface=None  automatic_assignment=on  address_offset=hex2dec('00')  intf_name=''  intf_description=''  default_value=0  timing_constraint=None  locs_specified=off  LOCs={}  io_standard={}  inherit_from_input=off  hdl_port=on  dbl_ovrd=off  block_type=gatewayin
  transfer : xbsIndex_r4/Gateway In  gui_display_data_type=Fixed-point  arith_type=Unsigned  n_bits=32  bin_pt=0  preci_type=Single  exp_width=8  frac_width=24  rows=1  columns=1  quantization="Round  (unbiased: +/- Inf)"  overflow=Saturate  period=1/(0.5*R_RRC*R_HB*R_CICcomp*R_CIC*Rb)  UseAsADC=off  ADCChannel='1'  interface=AXI4-Lite  automatic_assignment=off  address_offset=40  intf_name=''  intf_description=''  default_value=0  timing_constraint=None  locs_specified=off  LOCs={}  io_standard={}  inherit_from_input=off  hdl_port=on  dbl_ovrd=off  block_type=gatewayin
  transfer_dec : xbsIndex_r4/Gateway In  gui_display_data_type=Fixed-point  arith_type=Unsigned  n_bits=32  bin_pt=0  preci_type=Single  exp_width=8  frac_width=24  rows=1  columns=1  quantization="Round  (unbiased: +/- Inf)"  overflow=Saturate  period=1/(0.5*R_RRC*R_HB*R_CICcomp*R_CIC*Rb)  UseAsADC=off  ADCChannel='1'  interface=AXI4-Lite  automatic_assignment=off  address_offset=52  intf_name=''  intf_description=''  default_value=0  timing_constraint=None  locs_specified=off  LOCs={}  io_standard={}  inherit_from_input=off  hdl_port=on  dbl_ovrd=off  block_type=gatewayin
  transfer_rrc : xbsIndex_r4/Gateway In  gui_display_data_type=Fixed-point  arith_type=Unsigned  n_bits=32  bin_pt=0  preci_type=Single  exp_width=8  frac_width=24  rows=1  columns=1  quantization="Round  (unbiased: +/- Inf)"  overflow=Saturate  period=1/(0.5*R_RRC*R_HB*R_CICcomp*R_CIC*Rb)  UseAsADC=off  ADCChannel='1'  interface=AXI4-Lite  automatic_assignment=off  address_offset=64  intf_name=''  intf_description=''  default_value=0  timing_constraint=None  locs_specified=off  LOCs={}  io_standard={}  inherit_from_input=off  hdl_port=on  dbl_ovrd=off  block_type=gatewayin
  transfer_sync : xbsIndex_r4/Gateway In  gui_display_data_type=Fixed-point  arith_type=Unsigned  n_bits=32  bin_pt=0  preci_type=Single  exp_width=8  frac_width=24  rows=1  columns=1  quantization="Round  (unbiased: +/- Inf)"  overflow=Saturate  period=1/(0.5*R_RRC*R_HB*R_CICcomp*R_CIC*Rb)  UseAsADC=off  ADCChannel='1'  interface=AXI4-Lite  automatic_assignment=off  address_offset=76  intf_name=''  intf_description=''  default_value=0  timing_constraint=None  locs_specified=off  LOCs={}  io_standard={}  inherit_from_input=off  hdl_port=on  dbl_ovrd=off  block_type=gatewayin
  tData_I_out : Outport
  tValid_I_out : Outport  Port=2
  tReady_I_out : Outport  Port=3
  tData_Q_out : Outport  Port=4
  tValid_Q_out : Outport  Port=5
  tReady_Q_out : Outport  Port=6
  reset_out : Outport  Port=7
  packsetsize_out : Outport  Port=8
  enable_out : Outport  Port=9
  auto_restart_out : Outport  Port=10
  transfer_out : Outport  Port=11
  packet_size_dec_out : Outport  Port=12
  autorestart_dec_out : Outport  Port=13
  transfer_dec_out : Outport  Port=14
  packet_size_rrc_out : Outport  Port=15
  autorestart_rrc_out : Outport  Port=16
  transfer_rrc_out : Outport  Port=17
  packet_size_sync_out : Outport  Port=18
  autorestart_sync_out : Outport  Port=19
  transfer_sync_out : Outport  Port=20
  wires:
  packetsize_in/1 -> PacketSizeRF/1
  PacketSizeRF/1 -> packsetsize_out/1
  reset_in/1 -> RxReset/1
  Slice1/1 -> reset_out/1
  dataI_in/1 -> s_I_axis_tdata/1
  Enable/1 -> Slice/1
  Slice/1 -> enable_out/1
  s_I_axis_tdata/1 -> tData_I_out/1
  RxReset/1 -> Slice1/1
  enable_in/1 -> Enable/1
  dataQ_in/1 -> s_Q_axis_tdata/1
  s_Q_axis_tdata/1 -> tData_Q_out/1
  tValid_in/1 -> s_I_axis_tvalid/1
  s_I_axis_tready/1 -> tReady_I_out/1
  tReady_I_in/1 -> s_I_axis_tready/1
  s_I_axis_tvalid/1 -> tValid_I_out/1
  s_Q_axis_tvalid/1 -> tValid_Q_out/1
  tReady_Q_in/1 -> s_Q_axis_tready/1
  s_Q_axis_tready/1 -> tReady_Q_out/1
  tValid_Q_in/1 -> s_Q_axis_tvalid/1
  auto_restart_in/1 -> auto_restart/1
  Slice2/1 -> auto_restart_out/1
  auto_restart/1 -> Slice2/1
  transfer/1 -> Slice3/1
  Slice3/1 -> transfer_out/1
  transfer_in/1 -> transfer/1
  packet_size_dec_in/1 -> PacketSize_dec/1
  PacketSize_dec/1 -> packet_size_dec_out/1
  auto_restart_dec/1 -> Slice4/1
  Slice4/1 -> autorestart_dec_out/1
  autorestart_dec_in/1 -> auto_restart_dec/1
  transfer__dec_in/1 -> transfer_dec/1
  Slice5/1 -> transfer_dec_out/1
  packet_size_rrc_in/1 -> PacketSize_rrc/1
  PacketSize_rrc/1 -> packet_size_rrc_out/1
  auto_restart_rrc/1 -> Slice6/1
  Slice6/1 -> autorestart_rrc_out/1
  autorestart_rrc_in/1 -> auto_restart_rrc/1
  transfer_rrc_in/1 -> transfer_rrc/1
  transfer_rrc/1 -> Slice7/1
  Slice7/1 -> transfer_rrc_out/1
  packet_size_sync_in/1 -> PacketSize_sync/1
  PacketSize_sync/1 -> packet_size_sync_out/1
  autorestart_sync_in/1 -> auto_restart_sync/1
  auto_restart_sync/1 -> Slice8/1
  Slice8/1 -> autorestart_sync_out/1
  Slice9/1 -> transfer_sync_out/1
  transfer_sync/1 -> Slice9/1
  transfer_sync_in/1 -> transfer_sync/1
  transfer_dec/1 -> Slice5/1

== system AXI_QPSK_Rx/Subsystem/Timing Synch1 ==
  note: LATE (I)
  note: LATE (Q)
  note: EARLY (I)
  note: EARLY (Q)
  note: ONTIME (I)
  note: ONTIME (Q)
  I_In : Inport
  Q_In : Inport  Port=2
  Valid_in : Inport  Port=3
  AddSub : xbsIndex_r4/AddSub  mode=Subtraction  use_carryin=off  use_carryout=off  en=off  latency=0  precision=Full  arith_type=Unsigned  n_bits=16  bin_pt=14  quantization=Truncate  overflow=Wrap  use_behavioral_HDL=off  hw_selection=Fabric  pipelined=off  dbl_ovrd=off  block_type=addsub
  AddSub1 : xbsIndex_r4/AddSub  mode=Subtraction  use_carryin=off  use_carryout=off  en=off  latency=0  precision=Full  arith_type=Unsigned  n_bits=16  bin_pt=14  quantization=Truncate  overflow=Wrap  use_behavioral_HDL=off  hw_selection=Fabric  pipelined=off  dbl_ovrd=off  block_type=addsub
  AddSub2 : xbsIndex_r4/AddSub  mode=Addition  use_carryin=off  use_carryout=off  en=off  latency=0  precision=Full  arith_type=Unsigned  n_bits=16  bin_pt=14  quantization=Truncate  overflow=Wrap  use_behavioral_HDL=off  hw_selection=Fabric  pipelined=off  dbl_ovrd=off  block_type=addsub
  Delay : xbsIndex_r4/Delay  rst=off  infoeditControl=Selection of Reset will increase slice count due to use of real FFs and instead of SRLs  en=off  latency=OSR  reg_retiming=off  dbl_ovrd=off  block_type=delay
  Delay1 : xbsIndex_r4/Delay  rst=off  infoeditControl=Selection of Reset will increase slice count due to use of real FFs and instead of SRLs  en=off  latency=OSR  reg_retiming=off  dbl_ovrd=off  block_type=delay
  Delay10 : xbsIndex_r4/Delay  rst=off  infoeditControl=Selection of Reset will increase slice count due to use of real FFs and instead of SRLs  en=off  latency=1  reg_retiming=off  dbl_ovrd=off  block_type=delay
  Delay11 : xbsIndex_r4/Delay  rst=off  infoeditControl=Selection of Reset will increase slice count due to use of real FFs and instead of SRLs  en=off  latency=OSR/2  reg_retiming=off  dbl_ovrd=off  block_type=delay
  Delay12 : xbsIndex_r4/Delay  rst=off  infoeditControl=Selection of Reset will increase slice count due to use of real FFs and instead of SRLs  en=off  latency=1  reg_retiming=off  dbl_ovrd=off  block_type=delay
  Delay2 : xbsIndex_r4/Delay  rst=off  infoeditControl=Selection of Reset will increase slice count due to use of real FFs and instead of SRLs  en=off  latency=OSR/2  reg_retiming=off  dbl_ovrd=off  block_type=delay
  Delay6 : xbsIndex_r4/Delay  rst=off  infoeditControl=Selection of Reset will increase slice count due to use of real FFs and instead of SRLs  en=off  latency=OSR/2  reg_retiming=off  dbl_ovrd=off  block_type=delay
  Logical : xbsIndex_r4/Logical  logical_function=AND  inputs=2  en=off  latency=0  precision=Full  arith_type=Unsigned  n_bits=16  bin_pt=0  align_bp=on  dbl_ovrd=off  block_type=logical
  Loop Filter : Subsystem  mask(Loop Filter){Ka=Ka, Kb=Kb}
      mask prompts: Ka "Proportional gain (Ka)"; Kb "Integral gain (Kb)"
      mask help:
      | Filters the error signal generated by the Timing Error Detector.
      |
      | Key parameters are the gain of the proportional and integral branches.
  Mult1 : xbsIndex_r4/Mult  precision=User Defined  arith_type="Signed  (2's comp)"  n_bits=18  bin_pt=14  quantization=Truncate  overflow=Wrap  en=off  latency=0  use_behavioral_HDL=off  opt=Speed  use_embedded=on  optimum_pipeline=off  pipeline=on  dbl_ovrd=off  use_rpm=on  placement_style=Triangular  block_type=mult
  Mult2 : xbsIndex_r4/Mult  precision=User Defined  arith_type="Signed  (2's comp)"  n_bits=18  bin_pt=14  quantization=Truncate  overflow=Wrap  en=off  latency=0  use_behavioral_HDL=off  opt=Speed  use_embedded=on  optimum_pipeline=off  pipeline=on  dbl_ovrd=off  use_rpm=on  placement_style=Triangular  block_type=mult
  NCC : Subsystem  mask(Numerically Controlled Clock (NCC)){OSR=OSR, b=24}
      mask prompts: OSR "Oversampling ratio (nominal samples per symbol)"; b "Fractional bits"
      mask help: Creates strobes at a rate matching the symbol rate of the received data.
      mask init:
      | n = ceil(log2(OSR));
  Register : xbsIndex_r4/Register  init=0  rst=off  en=on  dbl_ovrd=off  block_type=register
  Register1 : xbsIndex_r4/Register  init=0  rst=off  en=on  dbl_ovrd=off  block_type=register
  Register2 : xbsIndex_r4/Register  init=0  rst=off  en=on  dbl_ovrd=off  block_type=register
  Terminator : Terminator
  Terminator1 : Terminator
  Terminator2 : Terminator
  Sample_Valid : Outport
  wires:
  Delay11/1 -> Register2/2, Register1/2, Delay12/1
  Delay/1 -> AddSub/2
  AddSub1/1 -> AddSub2/2
  Mult2/1 -> AddSub/1, Delay/1
  AddSub2/1 -> Register/1
  I_In/1 -> Delay6/1, Mult2/2, Mult2/1
  Q_In/1 -> Delay2/1, Mult1/1, Mult1/2
  Delay10/1 -> Loop Filter/2(En)
  Loop Filter/1(Error_Filt) -> NCC/1(Error_Filt)
  Delay2/1 -> Register2/1
  Delay6/1 -> Register1/1
  Mult1/1 -> Delay1/1, AddSub1/1
  AddSub/1 -> AddSub2/1
  Delay1/1 -> AddSub1/2
  Logical/1 -> Delay11/1, Register/2, Delay10/1
  Register/1 -> Loop Filter/1(Signal)
  Register2/1 -> Terminator2/1
  Delay12/1 -> Sample_Valid/1
  NCC/1(Strobe) -> Logical/1
  Valid_in/1 -> NCC/2(En), Logical/2
  NCC/2(Adj_Step) -> Terminator/1
  Register1/1 -> Terminator1/1
